simulink library "INP_IMU_Prep2"  (R2023b)
settings: Solver=VariableStepAuto  StartTime=0.0  StopTime=10.0  RelTol=1e-3
undefined symbols (not defined in the file): INP_c_TiSample_s, INP_IMU_p_AVehLatOfs_mps2, INP_IMU_p_AVehLatSca_na, INP_IMU_p_AVehLgtOfs_mps2, INP_IMU_p_AVehLgtSca_na, INP_IMU_p_AVehVertOfs_mps2, INP_IMU_p_AVehVertSca_na, INP_p_TiTau_s
libraries: VUT_lib x3
settings Model: Creator=blatak  LastModifiedBy=blatak

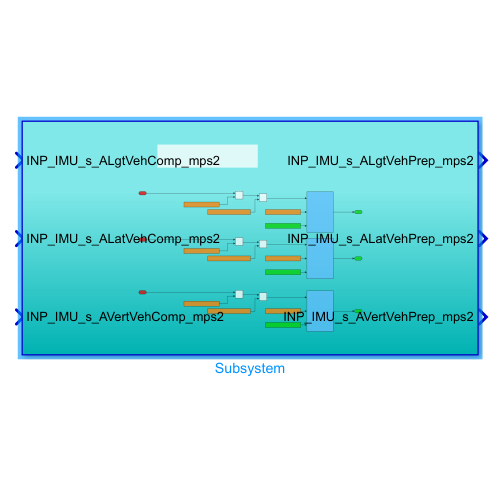
[thumbnail: Simulink's stored preview of the top-level diagram]
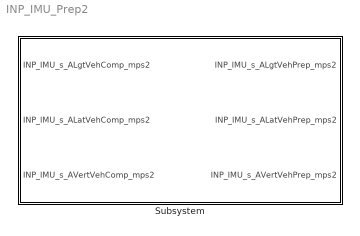
== system INP_IMU_Prep2 ==
  Subsystem : Subsystem  Description=Block transfers the value from electric quantitty to physical one (if needed), afterthat low pass filter is applied.

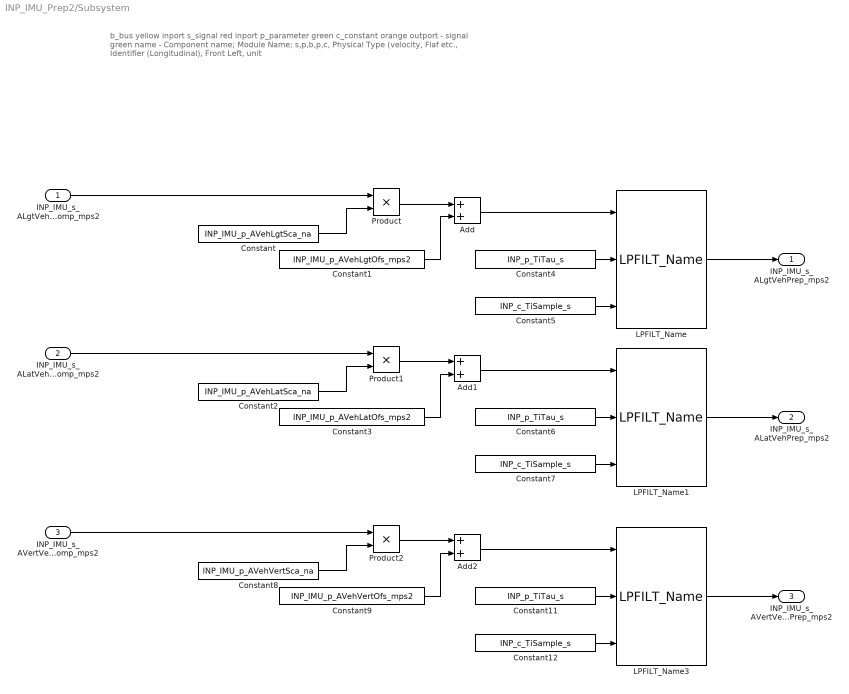
== system INP_IMU_Prep2/Subsystem ==
  note: b_bus yellow inport
      | s_signal red inport
      | p_parameter green
      | c_constant orange
      | outport - signal green
      | name - Component name; Module Name; s,p,b,p,c, Physical Type (velocity, Flaf etc., Identifier (Longitudinal), Front Left, unit
  INP_IMU_s_ALgtVehComp_mps2 : Inport  Description=IMU Comp Longitudinal acceleration - compensated value - from IMU position to cog
  INP_IMU_s_ALatVehComp_mps2 : Inport  Description=IMU Comp Lateral acceleration - compensated value - from IMU position to cog  Port=2
  INP_IMU_s_AVertVehComp_mps2 : Inport  Description=IMU Comp Vertical acceleration - compensated value - from IMU position to cog  Port=3
  Add : Sum
  Add1 : Sum
  Add2 : Sum
  Constant : Constant  Description=Scaling coefficient to recalculate the electric quantity to the physical one - longitudinal acceleration  Value=INP_IMU_p_AVehLgtSca_na
  Constant1 : Constant  Description=Offset to recalculate the electric quantity to the physical one - longitudinal acceleration  Value=INP_IMU_p_AVehLgtOfs_mps2
  Constant11 : Constant  Value=INP_p_TiTau_s
  Constant12 : Constant  Value=INP_c_TiSample_s
  Constant2 : Constant  Description=Scaling coefficient to recalculate the electric quantity to the physical one - lateral acceleration  Value=INP_IMU_p_AVehLatSca_na
  Constant3 : Constant  Description=Offset to recalculate the electric quantity to the physical one - lateral acceleration  Value=INP_IMU_p_AVehLatOfs_mps2
  Constant4 : Constant  Value=INP_p_TiTau_s
  Constant5 : Constant  Value=INP_c_TiSample_s
  Constant6 : Constant  Value=INP_p_TiTau_s
  Constant7 : Constant  Value=INP_c_TiSample_s
  Constant8 : Constant  Description=Scaling coefficient to recalculate the electric quantity to the physical one - vertical acceleration  Value=INP_IMU_p_AVehVertSca_na
  Constant9 : Constant  Description=Offset to recalculate the electric quantity to the physical one - vertical acceleration  Value=INP_IMU_p_AVehVertOfs_mps2
  LPFILT_Name : VUT_lib/LPFILT_Name  SystemSampleTime=-1  VariantActivationTime=update diagram  AllowFlexibleInterface=on  Latency=0  AutoFrameSizeCalculation=off
  LPFILT_Name1 : VUT_lib/LPFILT_Name  SystemSampleTime=-1  VariantActivationTime=update diagram  AllowFlexibleInterface=on  Latency=0  AutoFrameSizeCalculation=off
  LPFILT_Name3 : VUT_lib/LPFILT_Name  SystemSampleTime=-1  VariantActivationTime=update diagram  AllowFlexibleInterface=on  Latency=0  AutoFrameSizeCalculation=off
  Product : Product
  Product1 : Product
  Product2 : Product
  INP_IMU_s_ALgtVehPrep_mps2 : Outport  Description=IMU Prep Longitudinal acceleration - prepared value - scale, offset, filtering
  INP_IMU_s_ALatVehPrep_mps2 : Outport  Description=IMU Prep Lateral acceleration - prepared value - scale, offset, filtering  Port=2
  INP_IMU_s_AVertVehPrep_mps2 : Outport  Description=IMU Prep Vertical acceleration - prepared value - scale, offset, filtering  Port=3
  wires:
  LPFILT_Name3/1 -> INP_IMU_s_AVertVehPrep_mps2/1
  Add/1 -> LPFILT_Name/1
  Product1/1 -> Add1/1
  Product/1 -> Add/1
  Constant8/1 -> Product2/2
  Add1/1 -> LPFILT_Name1/1
  INP_IMU_s_ALatVehComp_mps2/1 -> Product1/1
  Constant/1 -> Product/2
  INP_IMU_s_ALgtVehComp_mps2/1 -> Product/1
  LPFILT_Name/1 -> INP_IMU_s_ALgtVehPrep_mps2/1
  Constant2/1 -> Product1/2
  Constant12/1 -> LPFILT_Name3/3
  Constant3/1 -> Add1/2
  Constant1/1 -> Add/2
  Constant9/1 -> Add2/2
  Product2/1 -> Add2/1
  LPFILT_Name1/1 -> INP_IMU_s_ALatVehPrep_mps2/1
  INP_IMU_s_AVertVehComp_mps2/1 -> Product2/1
  Constant11/1 -> LPFILT_Name3/2
  Constant6/1 -> LPFILT_Name1/2
  Constant5/1 -> LPFILT_Name/3
  Add2/1 -> LPFILT_Name3/1
  Constant7/1 -> LPFILT_Name1/3
  Constant4/1 -> LPFILT_Name/2
